simulink model "tqdtqr_rebuild_V3"  (R2021b)
settings: Solver=VariableStepAuto  StartTime=0.0  StopTime=10.0  RelTol=1e-3
undefined symbols (not defined in the file): ATQD_AfterTqMinGain_X_Deg, ATQD_APSCreepBaseTqD_X_kph, ATQD_APSCreepBaseTqD_Y_Deg, ATQD_APSCreepBaseTqR_X_kph, ATQD_APSCreepBaseTqR_Y_Deg, ATQD_APSCreepIterm_X_kph, ATQD_APSCreepIterm_Y_kph, ATQD_APSCreepPterm_X_kph, ATQD_APSCreepPterm_Y_kph, ATQD_APSDecReq_X_kph, ATQD_APSDecReq_Y_mps2, ATQD_APSDecReqCMD_X_kph, ATQD_APSDecReqTs_X_pct, ATQD_APSDecTimeGain_X_Deg, ATQD_APSDecTimeGain_Y_s, ATQD_APSReqLowSpd_X_Deg, ATQD_AutoHoldReleaseBPS_X_Deg, ATQD_AWDLoadTrqnsGain_X_kg, ATQD_AWDLoadTrqnsGain_Y_pct, ATQD_BOSEnBPSPosn_X_kph, ATQD_BOSMap_X_rpm, ATQD_BOSMap_Y_pct, ATQD_CreepBaseTqD_X_kph, ATQD_CreepBaseTqD_Y_Deg, ATQD_CreepBaseTqR_X_kph, ATQD_CreepBaseTqR_Y_Deg, ATQD_CreepBPSDisPosn_X_Deg, ATQD_CreepBPSDisPosnR_X_Deg, ATQD_CreepBPSEnPosn_X_Deg, ATQD_CreepBPSEnPosnR_X_Deg, ATQD_CreepDeltaTq_X_kph, ATQD_CreepIterm_X_kph, ATQD_CreepIterm_Y_kph, ATQD_CreepItermMaxLimit_X_pct, ATQD_CreepPreloadTime_X_kph, ATQD_CreepPreloadTq_X_kph, ATQD_CreepPreloadTq_Y_s, ATQD_CreepProtTq_X_Deg, ATQD_CreepPterm_X_kph, ATQD_CreepPterm_Y_kph, ATQD_CreepRrTqSpRat_X_rpm, ATQD_CreepRrTqSpRat_Y_Nm, ATQD_CreepTargetSpdD_X_pct, ATQD_CreepTargetSpdR_X_pct, ATQD_CreepUpLimitTq_X_rpm, ATQD_DecIneOPDHoldEnDelay_X_Deg, ATQD_DecIneOPDHoldEnDelay_Y_bar, ATQD_ECOTqMapD_X_rpm, ATQD_ECOTqMapD_Y_pct, ATQD_EMTqMapD_X_rpm, ATQD_EMTqMapD_Y_pct, ATQD_EOPDTqMapDCon_X_rpm, ATQD_EOPDTqMapDCon_Y_Deg, ATQD_EstInitVehWeight_X_c, ATQD_FAfterTqCMDGain_X_rpm, ATQD_FAfterTqCMDGain_Y_pct, ATQD_ForceLowSpd_X_Deg, ATQD_ForcePLimitSpd_X_Deg, ATQD_FrLossMAPLowV_X_rpm, ATQD_FrLossMAPLowV_Y_Nm ... (+949)
libraries: simulink x235, hcu_lib x208, tqr x63, tqd x6
(part 5 of 37)

== system tqdtqr_rebuild_V3/Main/Front//Rear first order input torque ==
  note: Front
  BInpConvert_outputs : Inport
  VTQD_AfterAvailableTqDemFr_Nm : Inport  Port=2
  VTQD_AfterAvailableTqDemRr_Nm : Inport  Port=3
  VTQR_FrFirstOrderOutTqDelay_Nm : Inport  Port=4
  VTQR_RrFirstOrderOutTqDelay_Nm : Inport  Port=5
  AND : Logic  AllPortsSameDT=off  OutDataTypeStr=boolean
  AND1 : Logic  AllPortsSameDT=off  OutDataTypeStr=boolean
  Bus Selector : BusSelector  OutputSignals=VTQR_RampTqCMDGain_c,VTQR_FrGearChange_flg,VTQR_FrTqZeroTrans_enum,VTQR_FrTqZeroTransLowBound_Nm,VTQR_FrTqZeroTransUpBound_Nm,VTQR_RrGearChange_flg,VTQR_RrTqZeroTrans_enum,VTQR_RrTqZeroTransLowBound_Nm,VTQR_RrTqZeroTransUpBound_Nm
  Constant{1,8,13..14} (4 alike) : Constant  Value=ZERO_FLOAT
  Constant10 : Constant  Value=ENUM_TQZEROTRANS_NOZEROTRANS
  Constant11 : Constant  Value=KTQR_NewRampArchSW_flg
  Constant12 : Constant  Value=ONE_FLOAT
  Constant2 : Constant  Value=KTQR_GearChangeTqSW_flg
  Constant3 : Constant  Value=ENUM_TQZEROTRANS_NOZEROTRANS
  Constant4 : Constant  Value=KTQR_NewRampArchSW_flg
  Constant5 : Constant  Value=ONE_FLOAT
  Constant6 : Constant  Value=ZERO_INT
  Constant7 : Constant  Value=ZERO_INT
  Constant9 : Constant  Value=KTQR_GearChangeTqSW_flg
  Product : Product
  Product1 : Product
  Relational Operator : RelationalOperator  Operator===  OutDataTypeStr=boolean  RndMeth=Simplest
  Relational Operator{1,3,6,8} (4 alike) : RelationalOperator  OutDataTypeStr=boolean  RndMeth=Simplest
  Relational Operator2 : RelationalOperator  Operator=<=  OutDataTypeStr=boolean  RndMeth=Simplest
  Relational Operator4 : RelationalOperator  Operator=<  OutDataTypeStr=boolean  RndMeth=Simplest
  Relational Operator5 : RelationalOperator  Operator===  OutDataTypeStr=boolean  RndMeth=Simplest
  Relational Operator7 : RelationalOperator  Operator=<=  OutDataTypeStr=boolean  RndMeth=Simplest
  Relational Operator9 : RelationalOperator  Operator=<  OutDataTypeStr=boolean  RndMeth=Simplest
  Switch{,1..2,7..9} (6 alike) : Switch  Criteria=u2 ~= 0
  Switch{3..6,10..13} (8 alike) : Switch  Criteria=u2 > Threshold
  VTQR_FrFirstOrderInpTq_Nm : Outport
  VTQR_RrFirstOrderInpTq_Nm : Outport  Port=2
  wires:
  Switch6/1 -> Switch1/1
  [VTQD_AfterAvailableTqDemFr_Nm] -> Relational Operator3/1
  [VTQR_FrTqZeroTransUpBound_Nm] -> Switch6/3
  [VTQD_AfterAvailableTqDemFr_Nm] -> Product/1
  Switch4/1 -> Product/2
  Constant7/1 -> Relational Operator4/2
  Relational Operator4/1 -> Switch6/2
  Constant5/1 -> Switch4/3
  Switch/1 -> Switch3/3
  [VTQD_AfterAvailableTqDemFr_Nm] -> Relational Operator4/1
  [VTQR_FrActRampTqDem_Nm] -> Switch2/3
  Constant6/1 -> Relational Operator3/2
  [VTQR_FrTqZeroTrans_enum] -> Relational Operator/1
  Relational Operator3/1 -> Switch5/2
  [VTQR_FrTqZeroTransLowBound_Nm] -> Switch5/3
  [VTQR_FrTqZeroTransUpBound_Nm] -> Switch5/1
  [VTQR_FrActRampTqDem_Nm] -> Switch/1
  Switch5/1 -> Switch2/1
  [VTQR_FrTqZeroTransLowBound_Nm] -> Switch6/1
  Constant2/1 -> AND/2
  [VTQR_FrTqZeroTransLowBound_Nm] -> Relational Operator2/2
  Relational Operator/1 -> Switch/2
  [VTQR_RampTqCMDGain_c] -> Switch4/1
  Switch1/1 -> Switch/3
  Constant4/1 -> Switch4/2
  [VTQR_FrGearChange_flg] -> AND/1
  AND/1 -> Switch3/2
  Product/1 -> [VTQR_FrActRampTqDem_Nm]  "VTQR_FrActRampTqDem_Nm"
  Constant1/1 -> Switch3/1
  [VTQR_FrFirstOrderOutTqDelay_Nm] -> Relational Operator2/1
  Relational Operator2/1 -> Switch2/2
  Switch2/1 -> Switch1/3
  [VTQR_FrTqZeroTransUpBound_Nm] -> Relational Operator1/2
  Switch3/1 -> [VTQR_FrFirstOrderInpTq_Nm]  "VTQR_FrFirstOrderInpTq_Nm"
  Constant3/1 -> Relational Operator/2
  Relational Operator1/1 -> Switch1/2
  [VTQR_FrFirstOrderOutTqDelay_Nm] -> Relational Operator1/1
  VTQD_AfterAvailableTqDemFr_Nm/1 -> [VTQD_AfterAvailableTqDemFr_Nm]
  VTQD_AfterAvailableTqDemRr_Nm/1 -> [VTQD_AfterAvailableTqDemRr_Nm]
  BInpConvert_outputs/1 -> Bus Selector/1
  Bus Selector/1 -> [VTQR_RampTqCMDGain_c]  "<VTQR_RampTqCMDGain_c>"
  Bus Selector/2 -> [VTQR_FrGearChange_flg]  "<VTQR_FrGearChange_flg>"
  Bus Selector/3 -> [VTQR_FrTqZeroTrans_enum]  "<VTQR_FrTqZeroTrans_enum>"
  Bus Selector/4 -> [VTQR_FrTqZeroTransLowBound_Nm]  "<VTQR_FrTqZeroTransLowBound_Nm>"
  Bus Selector/5 -> [VTQR_FrTqZeroTransUpBound_Nm]  "<VTQR_FrTqZeroTransUpBound_Nm>"
  [VTQR_RrGearChange_flg] -> AND1/1
  Relational Operator7/1 -> Switch9/2
  [VTQR_RrFirstOrderOutTqDelay_Nm] -> Relational Operator6/1
  [VTQR_RrTqZeroTrans_enum] -> Relational Operator5/1
  [VTQR_RrTqZeroTransUpBound_Nm] -> Relational Operator6/2
  Switch8/1 -> Switch7/3
  Constant10/1 -> Relational Operator5/2
  [VTQR_RrActRampTqDem_Nm] -> Switch9/3
  [VTQD_AfterAvailableTqDemRr_Nm] -> Relational Operator8/1
  Switch13/1 -> Switch8/1
  [VTQR_RrTqZeroTransUpBound_Nm] -> Switch13/3
  Relational Operator9/1 -> Switch13/2
  Constant12/1 -> Switch11/3
  Switch12/1 -> Switch9/1
  Constant14/1 -> Relational Operator9/2
  Constant13/1 -> Relational Operator8/2
  Relational Operator5/1 -> Switch7/2
  [VTQR_RrTqZeroTransLowBound_Nm] -> Switch13/1
  Constant9/1 -> AND1/2
  Constant8/1 -> Switch10/1
  [VTQR_RrTqZeroTransUpBound_Nm] -> Switch12/1
  Switch11/1 -> Product1/2
  [VTQR_RampTqCMDGain_c] -> Switch11/1
  [VTQD_AfterAvailableTqDemRr_Nm] -> Relational Operator9/1
  Relational Operator6/1 -> Switch8/2
  Relational Operator8/1 -> Switch12/2
  [VTQR_RrActRampTqDem_Nm] -> Switch7/1
  [VTQR_RrTqZeroTransLowBound_Nm] -> Switch12/3
  Constant11/1 -> Switch11/2
  [VTQD_AfterAvailableTqDemRr_Nm] -> Product1/1
  Switch10/1 -> [VTQR_RrFirstOrderInpTq_Nm]  "VTQR_RrFirstOrderInpTq_Nm"
  Switch7/1 -> Switch10/3
  Product1/1 -> [VTQR_RrActRampTqDem_Nm]  "VTQR_RrActRampTqDem_Nm"
  [VTQR_RrFirstOrderOutTqDelay_Nm] -> Relational Operator7/1
  AND1/1 -> Switch10/2
  [VTQR_RrTqZeroTransLowBound_Nm] -> Relational Operator7/2
  Switch9/1 -> Switch8/3
  Bus Selector/6 -> [VTQR_RrGearChange_flg]  "<VTQR_RrGearChange_flg>"
  Bus Selector/7 -> [VTQR_RrTqZeroTrans_enum]  "<VTQR_RrTqZeroTrans_enum>"
  Bus Selector/8 -> [VTQR_RrTqZeroTransLowBound_Nm]  "<VTQR_RrTqZeroTransLowBound_Nm>"
  Bus Selector/9 -> [VTQR_RrTqZeroTransUpBound_Nm]  "<VTQR_RrTqZeroTransUpBound_Nm>"
  [VTQR_FrFirstOrderInpTq_Nm] -> VTQR_FrFirstOrderInpTq_Nm/1
  [VTQR_RrFirstOrderInpTq_Nm] -> VTQR_RrFirstOrderInpTq_Nm/1
  VTQR_RrFirstOrderOutTqDelay_Nm/1 -> [VTQR_RrFirstOrderOutTqDelay_Nm]
  VTQR_FrFirstOrderOutTqDelay_Nm/1 -> [VTQR_FrFirstOrderOutTqDelay_Nm]

== system tqdtqr_rebuild_V3/Main/Front//Rear ramp enable judge ==
  note: Rear final torque
  note: Front final torque
  BSCPIn_outputs : Inport
  BInpConvert_outputs : Inport  Port=2
  VTQR_RampFEDUWhlTqReq_Nm : Inport  Port=3
  VTQD_AfterAvailableTqDemFr_Nm : Inport  Port=4
  VTQR_RampREDUWhlTqReq_Nm : Inport  Port=5
  VTQD_AfterAvailableTqDemRr_Nm : Inport  Port=6
  Add : Sum
  Add1 : Sum
  Bus Selector : BusSelector  OutputSignals=VVMC_ADASForceIdle_flg
  Bus Selector1 : BusSelector  OutputSignals=VTQD_LoSpdBrkCtrl_flg,VTQR_RampTqCMDGain_c,VTQR_ActFEDUTqUpLimit_Nm,VTQR_ActFEDUTqLowLimit_Nm,VTQD_FEDUWhlTqBRegen_Nm,VTQD_REDUWhlTqBRegen_Nm,VTQR_ActREDUTqUpLimit_Nm,VTQR_ActREDUTqLowLimit_Nm
  Constant : Constant  Value=TRUE
  Constant1 : Constant  Value=FALSE
  Constant10 : Constant  Value=ONE_INT
  Constant12 : Constant  Value=ONE_INT
  Constant13 : Constant  Value=KTQR_NewRampArchSW_flg
  Constant2 : Constant  Value=TRUE
  Constant3 : Constant  Value=FALSE
  Constant9 : Constant  Value=KTQR_NewRampArchSW_flg
  Logical Operator1 : Logic  Operator=OR  AllPortsSameDT=off  OutDataTypeStr=boolean
  Logical Operator2 : Logic  Operator=OR  AllPortsSameDT=off  OutDataTypeStr=boolean
  Product : Product
  Product1 : Product
  Saturation Dynamic : simulink/Discontinuities/Saturation Dynamic  OutMin=[]  OutMax=[]  OutDataTypeStr=Inherit: Same as second input  OutDataType=fixdt(1, 16)  OutScaling=2^-10  DoSatur=off
  Saturation Dynamic1 : simulink/Discontinuities/Saturation Dynamic  OutMin=[]  OutMax=[]  OutDataTypeStr=Inherit: Same as second input  OutDataType=fixdt(1, 16)  OutScaling=2^-10  DoSatur=off
  Switch{,1..3} (4 alike) : Switch  Criteria=u2 ~= 0
  Switch10 : Switch  Criteria=u2 > Threshold
  Switch11 : Switch  Criteria=u2 > Threshold
  VTQR_ActualFEDUWhlTqReq_Nm : Outport
  VTQR_NoABSFEDUWhlTqReq_Nm : Outport  Port=2
  VTQR_ActualREDUWhlTqReq_Nm : Outport  Port=3
  VTQR_NoABSREDUWhlTqReq_Nm : Outport  Port=4
  wires:
  Product/1 -> Switch/3
  Constant1/1 -> Switch2/1
  [VTQD_LoSpdBrkCtrl_flg] -> Logical Operator1/2
  Switch2/1 -> Switch/2  "VTQR_FrRampEnable_flg"
  [VINP_ADASForceIdle_flg] -> Logical Operator1/1
  Constant9/1 -> Switch10/2
  Switch10/1 -> Product/2
  [VTQR_ActFEDUTqLowLimit_Nm] -> Saturation Dynamic/3
  Switch/1 -> Saturation Dynamic/2
  Constant/1 -> Switch2/3
  [VTQR_ActFEDUTqUpLimit_Nm] -> Saturation Dynamic/1
  Add/1 -> VTQR_ActualFEDUWhlTqReq_Nm/1  "VTQR_ActualFEDUWhlTqReq_Nm"
  [VTQD_FEDUWhlTqBRegen_Nm] -> Add/1
  Logical Operator1/1 -> Switch2/2
  [VTQR_RampFEDUWhlTqReq_Nm] -> Switch/1
  [VTQR_RampTqCMDGain_c] -> Switch10/1
  Saturation Dynamic/1 -> Add/2, VTQR_NoABSFEDUWhlTqReq_Nm/1  "VTQR_NoABSFEDUWhlTqReq_Nm"
  [VTQD_AfterAvailableTqDemFr_Nm] -> Product/1
  BSCPIn_outputs/1 -> Bus Selector/1
  BInpConvert_outputs/1 -> Bus Selector1/1
  Bus Selector/1 -> [VINP_ADASForceIdle_flg]  "<VVMC_ADASForceIdle_flg>"
  Bus Selector1/1 -> [VTQD_LoSpdBrkCtrl_flg]  "<VTQD_LoSpdBrkCtrl_flg>"
  VTQR_RampFEDUWhlTqReq_Nm/1 -> [VTQR_RampFEDUWhlTqReq_Nm]
  VTQD_AfterAvailableTqDemFr_Nm/1 -> [VTQD_AfterAvailableTqDemFr_Nm]
  Bus Selector1/2 -> [VTQR_RampTqCMDGain_c]  "<VTQR_RampTqCMDGain_c>"
  Bus Selector1/3 -> [VTQR_ActFEDUTqUpLimit_Nm]  "<VTQR_ActFEDUTqUpLimit_Nm>"
  Bus Selector1/4 -> [VTQR_ActFEDUTqLowLimit_Nm]  "<VTQR_ActFEDUTqLowLimit_Nm>"
  Bus Selector1/5 -> [VTQD_FEDUWhlTqBRegen_Nm]  "<VTQD_FEDUWhlTqBRegen_Nm>"
  [VTQR_ActREDUTqLowLimit_Nm] -> Saturation Dynamic1/3
  [VINP_ADASForceIdle_flg] -> Logical Operator2/1
  [VTQD_AfterAvailableTqDemRr_Nm] -> Product1/1
  Switch1/1 -> Saturation Dynamic1/2
  Constant3/1 -> Switch3/1
  Product1/1 -> Switch1/3
  Constant2/1 -> Switch3/3
  [VTQR_RampREDUWhlTqReq_Nm] -> Switch1/1
  Saturation Dynamic1/1 -> VTQR_NoABSREDUWhlTqReq_Nm/1, Add1/2  "VTQR_NoABSREDUWhlTqReq_Nm"
  Switch11/1 -> Product1/2
  Constant13/1 -> Switch11/2
  [VTQR_RampTqCMDGain_c] -> Switch11/1
  [VTQR_ActREDUTqUpLimit_Nm] -> Saturation Dynamic1/1
  Logical Operator2/1 -> Switch3/2
  Switch3/1 -> Switch1/2  "VTQR_RrRampEnable_flg"
  Constant12/1 -> Switch11/3
  Add1/1 -> VTQR_ActualREDUWhlTqReq_Nm/1  "VTQR_ActualREDUWhlTqReq_Nm"
  [VTQD_LoSpdBrkCtrl_flg] -> Logical Operator2/2
  [VTQD_REDUWhlTqBRegen_Nm] -> Add1/1
  VTQR_RampREDUWhlTqReq_Nm/1 -> [VTQR_RampREDUWhlTqReq_Nm]
  VTQD_AfterAvailableTqDemRr_Nm/1 -> [VTQD_AfterAvailableTqDemRr_Nm]
  Bus Selector1/6 -> [VTQD_REDUWhlTqBRegen_Nm]  "<VTQD_REDUWhlTqBRegen_Nm>"
  Bus Selector1/7 -> [VTQR_ActREDUTqUpLimit_Nm]  "<VTQR_ActREDUTqUpLimit_Nm>"
  Bus Selector1/8 -> [VTQR_ActREDUTqLowLimit_Nm]  "<VTQR_ActREDUTqLowLimit_Nm>"
  Constant10/1 -> Switch10/3

== system tqdtqr_rebuild_V3/Main/Inverse and turn to motor torque ==
  note: Rear
  note: Front
  BSCPIn_outputs : Inport
  BInpConvert_outputs : Inport  Port=2
  VTQR_ActualFEDUWhlTqReq_Nm : Inport  Port=3
  VTQR_ActualREDUWhlTqReq_Nm : Inport  Port=4
  AND : Logic  AllPortsSameDT=off  OutDataTypeStr=boolean
  AND1 : Logic  AllPortsSameDT=off  OutDataTypeStr=boolean
  AND{2..5} (4 alike) : Logic  Inputs=3  AllPortsSameDT=off  OutDataTypeStr=boolean
  AND6 : Logic  Operator=OR  AllPortsSameDT=off  OutDataTypeStr=boolean
  AND7 : Logic  Operator=OR  AllPortsSameDT=off  OutDataTypeStr=boolean
  Bus Selector : BusSelector  OutputSignals=VVMC_ADASActive_flg
  Bus Selector1 : BusSelector  OutputSignals=VTQR_FrGearChange_flg,VTQD_PreLoadPreEn_flg,VTQD_PreLoadHold_flg,VTQD_GearActualPosn_enum,VTQR_RrGearChange_flg
  Constant : Constant  Value=KTQR_FrAbsoluteMTTqDir_flg
  Constant1 : Constant  Value=ENUM_GEARACTUALPOSN_R
  Constant{10..11,14,17} (4 alike) : Constant  Value=ONE_FLOAT
  Constant{8,12,15,18} (4 alike) : Constant  Value=ZERO_FLOAT
  Constant{9,13,16,19} (4 alike) : Constant  Value=MINUSONE_FLOAT
  Constant2 : Constant  Value=ENUM_GEARACTUALPOSN_R
  Constant21 : Constant  Value=KTQR_GearChangeTqSW_flg
  Constant23 : Constant  Value=KTQR_GearChangeTqDSW_flg
  Constant24 : Constant  Value=KTQR_GearChangeTqSW_flg
  Constant25 : Constant  Value=KTQR_GearChangeTqDSW_flg
  Constant26 : Constant  Value=KTQR_NewRampArchSW_flg
  Constant27 : Constant  Value=KTQR_NewRampArchSW_flg
  Constant3 : Constant  Value=KTQD_RrTMTotalGearRatio_gain
  Constant4 : Constant  Value=KTQR_RrAbsoluteMTTqDir_flg
  Constant5 : Constant  Value=KTQD_FrTMTotalGearRatio_gain
  Constant6 : Constant  Value=KTQR_FrTMGearEff_c
  Constant7 : Constant  Value=KTQR_RrTMGearEff_c
  Delay{,1..3} (4 alike) : Delay  DelayLength=1
  Divide : Product  Inputs=*//
  Divide1 : Product  Inputs=*//
  Equal : RelationalOperator  Operator===  OutDataTypeStr=boolean  RndMeth=Simplest
  Equal1 : RelationalOperator  Operator===  OutDataTypeStr=boolean  RndMeth=Simplest
  LiuZgSwitch1 : Switch  Criteria=u2 ~= 0  Threshold=0.5
      settings: AttributesFormatString=<%<Criteria>>
  LiuZgSwitch8 : Switch  Criteria=u2 ~= 0  Threshold=0.5
      settings: AttributesFormatString=<%<Criteria>>
  NOT{,1..3} (4 alike) : Logic  Operator=NOT  AllPortsSameDT=off  OutDataTypeStr=boolean
  Product{,1..3} (4 alike) : Product
  Relational Operator : RelationalOperator  Operator=>  OutDataTypeStr=boolean  RndMeth=Simplest
  Relational Operator1 : RelationalOperator  Operator=<  OutDataTypeStr=boolean  RndMeth=Simplest
  Relational Operator2 : RelationalOperator  Operator=<  OutDataTypeStr=boolean  RndMeth=Simplest
  Relational Operator3 : RelationalOperator  Operator=>  OutDataTypeStr=boolean  RndMeth=Simplest
  Switch{,1..3} (4 alike) : Switch  Criteria=u2 ~= 0
  Switch{4..9} (6 alike) : Switch  Criteria=u2 > Threshold
  VTQR_FrTMTqReq_Nm : Outport
  VTQR_RrTMTqReq_Nm : Outport  Port=2
  wires:
  AND7/1 -> Switch5/2
  [VTQR_FrGearChange_flg] -> Switch5/1
  [VTQR_ActualFEDUWhlTqReq_Nm] -> Product/2
  [VTQD_PreLoadPreEn_flg] -> AND3/2
  [VVMC_ADASActive_flg] -> AND7/2
  Switch8/1 -> Divide/1  "VTQR_InitFEDUWhlTqReq_Nm"
  [VTQD_PreLoadHold_flg] -> NOT1/1
  AND/1 -> LiuZgSwitch8/2
  Constant/1 -> AND/1
  NOT1/1 -> AND3/3
  Switch1/1 -> Product1/1
  Switch5/1 -> Switch1/2
  NOT/1 -> AND2/3
  LiuZgSwitch8/1 -> Switch8/3
  Product/1 -> LiuZgSwitch8/1
  AND3/1 -> Switch5/3
  Constant26/1 -> Switch8/2
  Product1/1 -> LiuZgSwitch8/3
  Constant21/1 -> Switch4/2
  [VTQR_ActualFEDUWhlTqReq_Nm] -> Switch8/1
  Equal/1 -> AND/2
  Switch4/1 -> Switch/2
  Switch/1 -> Product/1
  Constant11/1 -> Switch1/3
  [VTQD_GearActualPosn_enum] -> Equal/1
  Constant10/1 -> Switch/1
  Constant9/1 -> Switch/3
  Constant1/1 -> Equal/2
  Constant6/1 -> Divide/3
  Relational Operator1/1 -> AND3/1
  Relational Operator/1 -> AND2/1
  [VTQR_FrGearChange_flg] -> Switch4/1
  Delay1/1 -> Relational Operator1/1
  Divide/1 -> [VTQR_FrTMTqReq_Nm]  "VTQR_FrTMTqReq_Nm"
  AND2/1 -> Switch4/3
  [VTQR_ActualFEDUWhlTqReq_Nm] -> Product1/2
  Delay/1 -> Relational Operator/1
  [VTQR_FrTMTqReq_Nm] -> Delay/1
  Constant12/1 -> Relational Operator1/2
  Constant8/1 -> Relational Operator/2
  [VTQD_PreLoadHold_flg] -> NOT/1
  Constant23/1 -> AND7/1
  [VTQR_FrTMTqReq_Nm] -> Delay1/1
  Constant13/1 -> Switch1/1
  [VTQD_PreLoadPreEn_flg] -> AND2/2
  Constant5/1 -> Divide/2
  [VVMC_ADASActive_flg] -> AND6/2
  AND4/1 -> Switch7/3
  Switch6/1 -> Switch3/2
  [VTQR_ActualREDUWhlTqReq_Nm] -> Product3/2
  Delay2/1 -> Relational Operator2/1
  Constant24/1 -> Switch6/2
  Constant7/1 -> Divide1/3
  LiuZgSwitch1/1 -> Switch9/3
  [VTQR_RrTMTqReq_Nm] -> Delay2/1
  [VTQR_RrGearChange_flg] -> Switch7/1
  [VTQR_RrGearChange_flg] -> Switch6/1
  Constant27/1 -> Switch9/2
  [VTQD_GearActualPosn_enum] -> Equal1/1
  AND5/1 -> Switch6/3
  AND6/1 -> Switch7/2
  Switch7/1 -> Switch2/2
  [VTQD_PreLoadHold_flg] -> NOT3/1
  NOT3/1 -> AND5/3
  Constant15/1 -> Relational Operator2/2
  Constant19/1 -> Switch3/3
  Constant16/1 -> Switch2/1
  Product3/1 -> LiuZgSwitch1/1
  [VTQR_RrTMTqReq_Nm] -> Delay3/1
  Delay3/1 -> Relational Operator3/1
  Constant3/1 -> Divide1/2
  Constant2/1 -> Equal1/2
  AND1/1 -> LiuZgSwitch1/2
  [VTQD_PreLoadPreEn_flg] -> AND4/2
  NOT2/1 -> AND4/3
  Constant14/1 -> Switch2/3
  [VTQR_ActualREDUWhlTqReq_Nm] -> Switch9/1
  Equal1/1 -> AND1/2
  [VTQR_ActualREDUWhlTqReq_Nm] -> Product2/2
  Constant4/1 -> AND1/1
  [VTQD_PreLoadHold_flg] -> NOT2/1
  Product2/1 -> LiuZgSwitch1/3
  Constant25/1 -> AND6/1
  Constant18/1 -> Relational Operator3/2
  Switch2/1 -> Product2/1
  Divide1/1 -> [VTQR_RrTMTqReq_Nm]  "VTQR_RrTMTqReq_Nm"
  Constant17/1 -> Switch3/1
  Relational Operator3/1 -> AND5/1
  Switch3/1 -> Product3/1
  [VTQD_PreLoadPreEn_flg] -> AND5/2
  Relational Operator2/1 -> AND4/1
  Switch9/1 -> Divide1/1  "VTQR_InitREDUWhlTqReq_Nm"
  BSCPIn_outputs/1 -> Bus Selector/1
  BInpConvert_outputs/1 -> Bus Selector1/1
  Bus Selector1/1 -> [VTQR_FrGearChange_flg]  "<VTQR_FrGearChange_flg>"
  Bus Selector1/2 -> [VTQD_PreLoadPreEn_flg]  "<VTQD_PreLoadPreEn_flg>"
  Bus Selector1/3 -> [VTQD_PreLoadHold_flg]  "<VTQD_PreLoadHold_flg>"
  VTQR_ActualFEDUWhlTqReq_Nm/1 -> [VTQR_ActualFEDUWhlTqReq_Nm]
  VTQR_ActualREDUWhlTqReq_Nm/1 -> [VTQR_ActualREDUWhlTqReq_Nm]
  Bus Selector1/4 -> [VTQD_GearActualPosn_enum]  "<VTQD_GearActualPosn_enum>"
  Bus Selector/1 -> [VVMC_ADASActive_flg]  "<VVMC_ADASActive_flg>"
  Bus Selector1/5 -> [VTQR_RrGearChange_flg]  "<VTQR_RrGearChange_flg>"
  [VTQR_FrTMTqReq_Nm] -> VTQR_FrTMTqReq_Nm/1
  [VTQR_RrTMTqReq_Nm] -> VTQR_RrTMTqReq_Nm/1

== system tqdtqr_rebuild_V3/Main/Tq Coordination ==
  note: Determine coordination torque
  BSCPIn_outputs : Inport
  BInpConvert_outputs : Inport  Port=2
  VTQD_DriverWhlTqDem_Nm : Inport  Port=3
  Bus Selector : BusSelector  OutputSignals=VTQD_NoSuitbleGear_flg,VTQD_PreLoadHold_flg,VTQD_TotalWhlTqCapMot_Nm,VTQD_TotalWhlTqCapGen_Nm,VTQD_ForceIdleTqReq_Nm
  Bus Selector1 : BusSelector  OutputSignals=VVMC_ADASActive_flg,VVMC_ADASWhlTqReq_Nm,VVMC_CruzActive_flg,VVMC_CruzWhlTqReq_Nm,VVMC_MSAActive_flg,VVMC_MSAWhlTqReq_Nm,VVMC_APSActive_flg,VVMC_ADASForceIdle_flg
  Constant3 : Constant  Value=KTQD_NewTotalCapTqSW_flg
  Constant5 : Constant  Value=KTQD_DriverTqDemN_Nm
  Saturation Dynamic : simulink/Discontinuities/Saturation Dynamic  OutMin=[]  OutMax=[]  OutDataTypeStr=Inherit: Same as second input  OutDataType=fixdt(1, 16)  OutScaling=2^-10  DoSatur=off
  Switch{,1..6,8} (8 alike) : Switch  Criteria=u2 ~= 0
      settings: AttributesFormatString=%<Criteria>
  VTQD_CoordTqDem_Nm : Outport
  wires:
  [VTQD_TotalWhlTqCapMot_Nm] -> Saturation Dynamic/1
  [VTQD_TotalWhlTqCapGen_Nm] -> Saturation Dynamic/3
  Saturation Dynamic/1 -> Switch/1
  Constant3/1 -> Switch/2
  BInpConvert_outputs/1 -> Bus Selector/1
  BSCPIn_outputs/1 -> Bus Selector1/1
  Bus Selector1/1 -> [VVMC_ADASActive_flg]  "<VVMC_ADASActive_flg>"
  Bus Selector1/2 -> [VVMC_ADASWhlTqReq_Nm]  "<VVMC_ADASWhlTqReq_Nm>"
  Bus Selector1/3 -> [VVMC_CruzActive_flg]  "<VVMC_CruzActive_flg>"
  Bus Selector1/4 -> [VVMC_CruzWhlTqReq_Nm]  "<VVMC_CruzWhlTqReq_Nm>"
  Bus Selector1/5 -> [VVMC_MSAActive_flg]  "<VVMC_MSAActive_flg>"
  Bus Selector1/6 -> [VVMC_MSAWhlTqReq_Nm]  "<VVMC_MSAWhlTqReq_Nm>"
  Bus Selector1/7 -> [VVMC_APSActive_flg]  "<VVMC_APSActive_flg>"
  VTQD_DriverWhlTqDem_Nm/1 -> [VTQD_DriverWhlTqDem_Nm]
  Bus Selector1/8 -> [VINP_ADASForceIdle_flg]  "<VVMC_ADASForceIdle_flg>"
  Bus Selector/2 -> [VTQD_PreLoadHold_flg]  "<VTQD_PreLoadHold_flg>"
  Bus Selector/3 -> [VTQD_TotalWhlTqCapMot_Nm]  "<VTQD_TotalWhlTqCapMot_Nm>"
  Bus Selector/4 -> [VTQD_TotalWhlTqCapGen_Nm]  "<VTQD_TotalWhlTqCapGen_Nm>"
  Switch/1 -> [VTQD_CoordTqDem_Nm]  "VTQD_CoordTqDem_Nm"
  Bus Selector/1 -> [VTQD_NoSuitbleGear_flg]  "<VTQD_NoSuitbleGear_flg>"
  [VTQD_NoSuitbleGear_flg] -> Switch1/2
  Switch1/1 -> [VTQD_WhlTqReqMerge_Nm]
  Constant5/1 -> Switch1/1
  Switch8/1 -> Switch1/3
  [VINP_ADASForceIdle_flg] -> Switch8/2
  Switch2/1 -> Switch8/3
  [VVMC_ADASActive_flg] -> Switch2/2
  [VTQD_PreLoadHold_flg] -> Switch3/2
  Switch3/1 -> Switch2/1
  [VVMC_ADASWhlTqReq_Nm] -> Switch3/3
  [VTQD_DriverWhlTqDem_Nm] -> Switch3/1
  Switch4/1 -> Switch2/3
  [VVMC_MSAActive_flg] -> Switch5/2
  [VVMC_MSAWhlTqReq_Nm] -> Switch5/1
  [VVMC_CruzWhlTqReq_Nm] -> Switch4/1
  [VVMC_CruzActive_flg] -> Switch4/2
  Switch5/1 -> Switch4/3
  Switch6/1 -> Switch5/3
  [VVMC_APSActive_flg] -> Switch6/2
  [VTQD_DriverWhlTqDem_Nm] -> Switch6/1
  [VTQD_DriverWhlTqDem_Nm] -> Switch6/3
  [VTQD_WhlTqReqMerge_Nm] -> Saturation Dynamic/2
  [VTQD_WhlTqReqMerge_Nm] -> Switch/3
  [VTQD_CoordTqDem_Nm] -> VTQD_CoordTqDem_Nm/1
  Bus Selector/5 -> [VTQD_ForceIdleTqReq_Nm]  "<VTQD_ForceIdleTqReq_Nm>"
  [VTQD_ForceIdleTqReq_Nm] -> Switch8/1

== system tqdtqr_rebuild_V3/Main/Tq Distribution ==
  note: Calculate Fr/Rr demand torque
  BSCPIn_outputs : Inport
  BInpConvert_outputs : Inport  Port=2
  TqCoordination_outputs : Inport  Port=3
  AND : Logic  Inputs=4  AllPortsSameDT=off  OutDataTypeStr=boolean
  AND1 : Logic  Inputs=4  AllPortsSameDT=off  OutDataTypeStr=boolean
  AND11 : Logic  Inputs=3  AllPortsSameDT=off  OutDataTypeStr=boolean
  AND{8..9,12,14} (4 alike) : Logic  AllPortsSameDT=off  OutDataTypeStr=boolean
  AND13 : Logic  Inputs=3  AllPortsSameDT=off  OutDataTypeStr=boolean
  Add : Sum
  Add1 : Sum  Inputs=+-
  Add2 : Sum
  Add3 : Sum  Inputs=+-
  Bus Selector : BusSelector  OutputSignals=VINP_RearAxlTrqReqDrv_Nm,VPMM_DrivetrainSelect_enum,VINP_RrPTCSActive_flg,VINP_FrPTCSActive_flg,VINP_FrntAxlTrqReqDrv_Nm
  Bus Selector1 : BusSelector  OutputSignals=VTQD_RockModePedTqFr_Nm,VTQD_RockModeTqLim_flg,VTQD_FrPreloadTq_Nm,VTQD_PreLoadHold_flg,VTQD_RockModePedTqRr_Nm,VTQD_RrPreloadTq_Nm,VTQD_NewDistFrWhlTq_Nm,VTQD_NewDistRrWhlTq_Nm,VTQD_FrEDUSpRat_rat,VTQD_RrEDUSpRat_rat
  Constant27 : Constant  Value=KTQD_RocModeTqCtrlSW_flg  VectorParams1D=off  SampleTime=-1
  Constant28 : Constant  Value=KTQD_RocModeTqCtrlSW_flg  VectorParams1D=off  SampleTime=-1
  Constant3 : Constant  Value=ENUM_DRIVETRAIN_AWD  VectorParams1D=off  SampleTime=-1
  Constant{34,37..38,41} (4 alike) : Constant  Value=KTQD_NewPrelaodSW_flg  VectorParams1D=off  SampleTime=-1
  Constant35 : Constant  Value=KTQD_NewWhlTqDistSW_flg  VectorParams1D=off  SampleTime=-1
  Constant36 : Constant  Value=KTQD_NewTotalCapTqSW_flg  VectorParams1D=off  SampleTime=-1
  Constant39 : Constant  Value=KTQD_NewWhlTqDistSW_flg  VectorParams1D=off  SampleTime=-1
  Constant4 : Constant  Value=ZERO_FLOAT  VectorParams1D=off  SampleTime=-1
  Constant40 : Constant  Value=KTQD_NewTotalCapTqSW_flg  VectorParams1D=off  SampleTime=-1
  Constant5 : Constant  Value=KTQD_RrTCSCompensateSW_flg  VectorParams1D=off  SampleTime=-1
  Constant6 : Constant  Value=ENUM_DRIVETRAIN_AWD  VectorParams1D=off  SampleTime=-1
  Constant7 : Constant  Value=ZERO_FLOAT  VectorParams1D=off  SampleTime=-1
  Constant8 : Constant  Value=KTQD_FrTCSCompensateSW_flg  VectorParams1D=off  SampleTime=-1
  Equal3 : RelationalOperator  Operator===  OutDataTypeStr=boolean  RndMeth=Simplest
  Equal4 : RelationalOperator  Operator===  OutDataTypeStr=boolean  RndMeth=Simplest
  NOT : Logic  Operator=NOT  AllPortsSameDT=off  OutDataTypeStr=boolean
  NOT2 : Logic  Operator=NOT  AllPortsSameDT=off  OutDataTypeStr=boolean
  Product1 : Product
  Product4 : Product
  Saturation : Saturate  UpperLimit=KTQD_TCSCompUpLimit_Nm  LowerLimit=ZERO_FLOAT
      settings: AttributesFormatString=%<UpperLimit>
  Saturation1 : Saturate  UpperLimit=KTQD_TCSCompUpLimit_Nm  LowerLimit=ZERO_FLOAT
      settings: AttributesFormatString=%<UpperLimit>
  Switch{,1,8..9,11..14} (8 alike) : Switch  Criteria=u2 ~= 0
      settings: AttributesFormatString=%<Criteria>
  VTQD_CoordWhlTqDemFr_Nm : Outport
  VTQD_CoordWhlTqDemRr_Nm : Outport  Port=2
  VTQD_CoordTqDemFr_Nm : Outport  Port=3
  VTQD_CoordTqDemRr_Nm : Outport  Port=4
  wires:
  BSCPIn_outputs/1 -> Bus Selector/1
  BInpConvert_outputs/1 -> Bus Selector1/1
  [VTQD_FrEDUSpRat_rat] -> Product4/1
  Constant36/1 -> AND11/2
  Constant34/1 -> AND12/2
  Constant35/1 -> AND11/3
  Switch1/1 -> Saturation1/1
  [VTQD_RockModeTqLim_flg] -> AND8/1
  Switch8/1 -> Add2/2, [VTQD_CoordTqDemFr_Nm]  "VTQD_CoordTqDemFr_Nm"
  [VTQD_CoordTqDem_Nm] -> Product4/2
  [VTQD_RockModePedTqFr_Nm] -> Switch8/1
  AND8/1 -> Switch8/2
  [VINP_RrPTCSActive_flg] -> AND1/2
  Constant8/1 -> AND1/4
  Constant7/1 -> Switch1/3
  Equal4/1 -> AND1/1
  [VTQD_CoordTqDemRr_Nm] -> Add3/1
  [VINP_FrPTCSActive_flg] -> NOT/1
  [VTQD_PreLoadHold_flg] -> AND12/1
  AND1/1 -> Switch1/2
  [VPMM_DrivetrainSelect_enum] -> Equal4/1
  Saturation1/1 -> Add2/1  "VTQD_FrTCSCompensateTq_Nm"
  AND12/1 -> Switch11/2
  Constant6/1 -> Equal4/2
  [VTQD_NewDistFrWhlTq_Nm] -> Switch12/1
  Switch11/1 -> Switch12/3
  NOT/1 -> AND1/3
  AND11/1 -> Switch12/2
  Add3/1 -> Switch1/1
  Constant27/1 -> AND8/2
  [VTQD_FrPreloadTq_Nm] -> Switch11/1
  [VINP_RearAxlTrqReqDrv_Nm] -> Add3/2
  Switch12/1 -> Switch8/3
  Product4/1 -> Switch11/3
  Constant37/1 -> AND11/1
  Constant39/1 -> AND13/3
  Constant40/1 -> AND13/2
  AND13/1 -> Switch14/2
  Product1/1 -> Switch13/3
  AND14/1 -> Switch13/2
  [VTQD_RrPreloadTq_Nm] -> Switch13/1
  Switch13/1 -> Switch14/3
  Switch9/1 -> Add/2, [VTQD_CoordTqDemRr_Nm]  "VTQD_CoordTqDemRr_Nm"
  Constant38/1 -> AND14/2
  Constant41/1 -> AND13/1
  [VTQD_NewDistRrWhlTq_Nm] -> Switch14/1
  Switch/1 -> Saturation/1
  Constant3/1 -> Equal3/2
  AND9/1 -> Switch9/2
  AND/1 -> Switch/2
  Constant28/1 -> AND9/2
  [VTQD_RockModeTqLim_flg] -> AND9/1
  NOT2/1 -> AND/3
  [VTQD_CoordTqDemFr_Nm] -> Add1/1
  Saturation/1 -> Add/1  "VTQD_RrTCSCompensateTq_Nm"
  [VPMM_DrivetrainSelect_enum] -> Equal3/1
  Add/1 -> [VTQD_CoordWhlTqDemRr_Nm]  "VTQD_CoordWhlTqDemRr_Nm"
  Constant5/1 -> AND/4
  Constant4/1 -> Switch/3
  Add1/1 -> Switch/1
  [VTQD_PreLoadHold_flg] -> AND14/1
  [VINP_RrPTCSActive_flg] -> NOT2/1
  Switch14/1 -> Switch9/3
  [VTQD_RrEDUSpRat_rat] -> Product1/1
  [VTQD_CoordTqDem_Nm] -> Product1/2
  [VINP_FrntAxlTrqReqDrv_Nm] -> Add1/2
  [VTQD_RockModePedTqRr_Nm] -> Switch9/1
  [VINP_FrPTCSActive_flg] -> AND/2
  Equal3/1 -> AND/1
  Bus Selector/1 -> [VINP_RearAxlTrqReqDrv_Nm]  "<VINP_RearAxlTrqReqDrv_Nm>"
  Bus Selector/2 -> [VPMM_DrivetrainSelect_enum]  "<VPMM_DrivetrainSelect_enum>"
  Bus Selector/3 -> [VINP_RrPTCSActive_flg]  "<VINP_RrPTCSActive_flg>"
  Bus Selector/4 -> [VINP_FrPTCSActive_flg]  "<VINP_FrPTCSActive_flg>"
  Bus Selector1/1 -> [VTQD_RockModePedTqFr_Nm]  "<VTQD_RockModePedTqFr_Nm>"
  Bus Selector1/2 -> [VTQD_RockModeTqLim_flg]  "<VTQD_RockModeTqLim_flg>"
  Bus Selector1/3 -> [VTQD_FrPreloadTq_Nm]  "<VTQD_FrPreloadTq_Nm>"
  Bus Selector1/4 -> [VTQD_PreLoadHold_flg]  "<VTQD_PreLoadHold_flg>"
  Bus Selector/5 -> [VINP_FrntAxlTrqReqDrv_Nm]  "<VINP_FrntAxlTrqReqDrv_Nm>"
  Bus Selector1/5 -> [VTQD_RockModePedTqRr_Nm]  "<VTQD_RockModePedTqRr_Nm>"
  Bus Selector1/6 -> [VTQD_RrPreloadTq_Nm]  "<VTQD_RrPreloadTq_Nm>"
  Add2/1 -> [VTQD_CoordWhlTqDemFr_Nm]  "VTQD_CoordWhlTqDemFr_Nm"
  Bus Selector1/7 -> [VTQD_NewDistFrWhlTq_Nm]  "<VTQD_NewDistFrWhlTq_Nm>"
  Bus Selector1/8 -> [VTQD_NewDistRrWhlTq_Nm]  "<VTQD_NewDistRrWhlTq_Nm>"
  TqCoordination_outputs/1 -> [VTQD_CoordTqDem_Nm]
  Bus Selector1/9 -> [VTQD_FrEDUSpRat_rat]  "<VTQD_FrEDUSpRat_rat>"
  Bus Selector1/10 -> [VTQD_RrEDUSpRat_rat]  "<VTQD_RrEDUSpRat_rat>"
  [VTQD_CoordWhlTqDemFr_Nm] -> VTQD_CoordWhlTqDemFr_Nm/1
  [VTQD_CoordWhlTqDemRr_Nm] -> VTQD_CoordWhlTqDemRr_Nm/1
  [VTQD_CoordTqDemFr_Nm] -> VTQD_CoordTqDemFr_Nm/1
  [VTQD_CoordTqDemRr_Nm] -> VTQD_CoordTqDemRr_Nm/1

== system tqdtqr_rebuild_V3/Output_Convert/Avaliable Torque ==
  note: Avaiable Torque for B-type Regen
  note: A-regen activation judgment
  BSCPIn_outputs : Inport
  BInpConvert_outputs : Inport  Port=2
  BMain_outputs : Inport  Port=3
  VTQD_DriverWhlTqDemFr_Nm : Inport  Port=4
  VTQD_DriverWhlTqDemRr_Nm : Inport  Port=5
  Bus Selector : BusSelector  OutputSignals=task_time_s,VVMC_ADASActive_flg,VINP_FrRegenAvailTq_Nm,VINP_RrRegenAvailTq_Nm,VINP_HVBattSOC_pct,VPMM_DrivetrainSelect_enum
  Bus Selector1 : BusSelector  OutputSignals=VTQD_TqSourceFr_enum,VTQD_TqSourceRr_enum,VTQD_CreepEnable_flg,VTQD_WhlTqCapGenFr_Nm,VTQD_WhlTqCapGenRr_Nm,VTQD_VehActSpd_kph,VTQD_GearActualPosn_enum
  Bus Selector2 : BusSelector  OutputSignals=VTQD_DriverWhlTqDem_Nm
  Constant{,4,7,37,44} (5 alike) : Constant  Value=FALSE
  Constant1 : Constant  Value=ENUM_TQSOURCE_CC
  Constant10 : Constant  Value=ENUM_TQSOURCE_APS
  Constant11 : Constant  Value=ENUM_TQSOURCE_CC
  Constant12 : Constant  Value=ENUM_TQSOURCE_APS
  Constant13 : Constant  Value=ENUM_TQSOURCE_ADAS
  Constant{14,17,20,33,48} (5 alike) : Constant  Value=ZERO_FLOAT
  Constant15 : Constant  Value=KTQD_AvailBrkRgnTqSpd_kph
  Constant18 : Constant  Value=KTQD_AvailBrkRgnTqSpd_kph
  Constant{3,6,8,38,45} (5 alike) : Constant  Value=TRUE
  Constant34 : Constant  Value=KTQD_AvailBRgnTqVSOC_pct
  Constant35 : Constant  Value=ENUM_GEARACTUALPOSN_N
  Constant36 : Constant  Value=ENUM_GEARACTUALPOSN_P
  Constant39 : Constant  Value=ENUM_DRIVETRAIN_RWD
  Constant40 : Constant  Value=ENUM_DRIVETRAIN_RWD
  Constant41 : Constant  Value=KTQD_BRgnPermDisDelay_s
  Constant42 : Constant  Value=ENUM_GEARACTUALPOSN_N
  Constant43 : Constant  Value=ENUM_GEARACTUALPOSN_P
  Constant46 : Constant  Value=ENUM_DRIVETRAIN_FWD
  Constant47 : Constant  Value=KTQD_BRgnPermDisDelay_s
  Constant49 : Constant  Value=KTQD_AvailBRgnTqVSOC_pct
  Constant50 : Constant  Value=ENUM_DRIVETRAIN_FWD
  Constant9 : Constant  Value=ENUM_TQSOURCE_ADAS
  Data Type Conversion : DataTypeConversion  OutDataTypeStr=single
  Data Type Conversion1 : DataTypeConversion  OutDataTypeStr=single
  DelayEnable : hcu_lib/Basic_Blocks/DelayEnable
  DelayEnable1 : hcu_lib/Basic_Blocks/DelayEnable
  Equal{,1..5,10..17} (14 alike) : RelationalOperator  Operator===  OutDataTypeStr=boolean  RndMeth=Simplest
  Gain : Gain  Gain=KTQD_FrTMTotalGearRatio_gain
  Gain1 : Gain  Gain=KTQD_RrTMTotalGearRatio_gain
  If : If  IfExpression=u1 ~= 0
  If Action Subsystem1 : tqd/TQD/TorqueDemand/TorqueModule/AvaliableTqLimit/If Action Subsystem1  SystemSampleTime=-1  VariantActivationTime=update diagram  Latency=0  AutoFrameSizeCalculation=off
  If Action Subsystem2 : tqd/TQD/TorqueDemand/TorqueModule/AvaliableTqLimit/If Action Subsystem2  SystemSampleTime=-1  VariantActivationTime=update diagram  Latency=0  AutoFrameSizeCalculation=off
  Logical Operator : Logic  Operator=OR  Inputs=7  AllPortsSameDT=off  OutDataTypeStr=boolean
  Logical Operator1 : Logic  AllPortsSameDT=off  OutDataTypeStr=boolean
  Logical Operator2 : Logic  Operator=NOT  AllPortsSameDT=off  OutDataTypeStr=boolean
  Max : MinMax  Function=max  Inputs=2
  Max1 : MinMax  Function=max  Inputs=2
  Merge : Merge
  Merge1 : Merge
  OR2 : Logic  Operator=OR  Inputs=3  AllPortsSameDT=off  OutDataTypeStr=boolean
  OR{3..6} (4 alike) : Logic  Operator=OR  AllPortsSameDT=off  OutDataTypeStr=boolean
  OR7 : Logic  Operator=OR  Inputs=3  AllPortsSameDT=off  OutDataTypeStr=boolean
  Relational Operator : RelationalOperator  Operator=<  OutDataTypeStr=boolean  RndMeth=Simplest
  Relational Operator1 : RelationalOperator  Operator=<=  OutDataTypeStr=boolean  RndMeth=Simplest
  Relational Operator2 : RelationalOperator  Operator=<=  OutDataTypeStr=boolean  RndMeth=Simplest
  Relational Operator{3..6} (4 alike) : RelationalOperator  OutDataTypeStr=boolean  RndMeth=Simplest
  Switch{,1,11..12} (4 alike) : Switch  Criteria=u2 > Threshold
  Switch2 : Switch  Criteria=u2 ~= 0
  Switch3 : Switch  Criteria=u2 ~= 0
  Switch4 : Switch  Criteria=u2 ~= 0
  VTQD_ARegenActive_flg : Outport
  VTQD_FrEDUAvailBrkRgnTq_Nm : Outport  Port=2
  VTQD_RrEDUAvailBrkRgnTq_Nm : Outport  Port=3
  VTQD_FrRgnDecrSta_flg : Outport  Port=4
  VTQD_RrRgnDecrSta_flg : Outport  Port=5
  VTQD_FrRgnPermSta_flg : Outport  Port=6
  VTQD_RrRgnPermSta_flg : Outport  Port=7
  wires:
  Logical Operator/1 -> Logical Operator2/1
  [VTQD_FrEDUAvailBrkRgnTq_Nm] -> Relational Operator3/1
  OR4/1 -> Switch11/2
  [VPMM_DrivetrainSelect_enum] -> Equal13/1
  [task_time_s] -> DelayEnable/3
  Constant20/1 -> Switch4/1
  Constant47/1 -> DelayEnable1/2
  Constant13/1 -> Equal4/2
  Constant45/1 -> Switch12/3
  Max1/1 -> Switch4/3
  Constant10/1 -> Equal2/2
  [VTQD_GearActualPosn_enum] -> Equal15/1
  [VTQD_DriverWhlTqDemRr_Nm] -> If Action Subsystem1/4
  [VPMM_DrivetrainSelect_enum] -> Equal12/1
  Constant9/1 -> Equal1/2
  Constant6/1 -> Switch1/3
  Constant18/1 -> Relational Operator2/2
  OR6/1 -> Switch12/2
  Constant44/1 -> Switch12/1
  Constant46/1 -> Equal16/2
  OR5/1 -> DelayEnable1/1
  Switch2/1 -> [VTQD_ARegenActive_flg]  "VTQD_ARegenActive_flg"
  [VVMC_ADASActive_flg] -> If Action Subsystem1/5
  [task_time_s] -> DelayEnable1/3
  Equal13/1 -> OR4/2
  Equal14/1 -> OR5/1
  Equal11/1 -> OR3/2
  [VTQD_AvailTqNoARgnFr_Nm] -> Merge/2
  Constant1/1 -> Equal/2
  DelayEnable/1 -> OR4/1
  Switch4/1 -> Data Type Conversion1/1
  OR3/1 -> DelayEnable/1
  Constant34/1 -> Relational Operator4/2
  [VTQD_GearActualPosn_enum] -> Equal11/1
  Constant41/1 -> DelayEnable/2
  [VTQD_RrEDUAvailBrkRgnTq_Nm] -> Relational Operator5/1
  Relational Operator6/1 -> OR7/2
  DelayEnable1/1 -> OR6/1
  [VPMM_DrivetrainSelect_enum] -> Equal17/1
  Constant40/1 -> Equal13/2
  Constant38/1 -> Switch11/3
  Relational Operator3/1 -> OR2/1
  [VTQD_TqSourceFr_enum] -> Equal/1
  [VTQD_GearActualPosn_enum] -> Equal10/1
  Constant37/1 -> Switch11/1
  Max/1 -> Switch3/3
  [VTQD_CreepEnable_flg] -> Logical Operator/7
  Equal10/1 -> OR3/1
  Constant35/1 -> Equal10/2
  [VTQD_AvailTqWithARgnFr_Nm] -> Merge/1
  Relational Operator4/1 -> OR2/2
  Constant33/1 -> Relational Operator3/2
  If/2 -> If Action Subsystem2/Action
  Constant/1 -> Switch/1
  Constant3/1 -> Switch/3
  [VINP_RrRegenAvailTq_Nm] -> Gain1/1
  Switch3/1 -> Data Type Conversion/1
  [VTQD_WhlTqCapGenFr_Nm] -> If Action Subsystem1/1
  [VTQD_DriverWhlTqDemFr_Nm] -> If Action Subsystem1/3
  If/1 -> If Action Subsystem1/Action
  Constant50/1 -> Equal17/2
  Logical Operator1/1 -> Switch2/2
  Relational Operator5/1 -> OR7/1
  Relational Operator1/1 -> Switch3/2
  Constant17/1 -> Switch3/1
  Equal15/1 -> OR5/2
  Equal1/1 -> Logical Operator/2
  Relational Operator/1 -> Logical Operator1/2
  [VTQD_TqSourceFr_enum] -> Equal2/1
  [VTQD_AvailTqWithARgnRr_Nm] -> Merge1/1
  [VTQD_TqSourceRr_enum] -> Equal3/1
  [VTQD_TqSourceRr_enum] -> Equal4/1
  [VTQD_TqSourceRr_enum] -> Equal5/1
  Equal4/1 -> Logical Operator/5
  Equal5/1 -> Logical Operator/6
  If Action Subsystem1/2 -> [VTQD_AvailTqWithARgnRr_Nm]
  Data Type Conversion/1 -> [VTQD_FrEDUAvailBrkRgnTq_Nm]  "VTQD_FrEDUAvailBrkRgnTq_Nm"
  [VTQD_DriverWhlTqDem_Nm] -> Relational Operator/1
  Constant15/1 -> Relational Operator1/2
  [VINP_HVBattSOC_pct] -> Relational Operator4/1
  Constant12/1 -> Equal5/2
  Gain/1 -> Max/1
  [VTQD_VehActSpd_kph] -> Relational Operator1/1
  If Action Subsystem2/1 -> [VTQD_AvailTqNoARgnFr_Nm]
  Data Type Conversion1/1 -> [VTQD_RrEDUAvailBrkRgnTq_Nm]  "VTQD_RrEDUAvailBrkRgnTq_Nm"
  Equal16/1 -> OR6/2
  Logical Operator2/1 -> Logical Operator1/1
  Equal3/1 -> Logical Operator/4
  Merge/1 -> Max/2
  OR7/1 -> Switch1/2
  If Action Subsystem1/1 -> [VTQD_AvailTqWithARgnFr_Nm]
  Gain1/1 -> Max1/1
  Equal2/1 -> Logical Operator/3
  [VTQD_TqSourceFr_enum] -> Equal1/1
  OR2/1 -> Switch/2
  [VTQD_AvailTqNoARgnRr_Nm] -> Merge1/2
  Relational Operator2/1 -> Switch4/2
  Constant42/1 -> Equal14/2
  [VINP_HVBattSOC_pct] -> Relational Operator6/1
  [VTQD_WhlTqCapGenRr_Nm] -> If Action Subsystem1/2
  Constant48/1 -> Relational Operator5/2
  Equal12/1 -> OR2/3
  Constant8/1 -> Switch2/1
  [VTQD_GearActualPosn_enum] -> Equal14/1
  [VTQD_WhlTqCapGenRr_Nm] -> If Action Subsystem2/2
  Merge1/1 -> Max1/2
  Constant4/1 -> Switch1/1
  If Action Subsystem2/2 -> [VTQD_AvailTqNoARgnRr_Nm]
  Constant36/1 -> Equal11/2
  [VPMM_DrivetrainSelect_enum] -> Equal16/1
  Constant49/1 -> Relational Operator6/2
  Constant14/1 -> Relational Operator/2
  [VTQD_ARegenActive_flg] -> If/1
  [VTQD_WhlTqCapGenFr_Nm] -> If Action Subsystem2/1
  Equal17/1 -> OR7/3
  Equal/1 -> Logical Operator/1
  Constant11/1 -> Equal3/2
  Constant43/1 -> Equal15/2
  Constant7/1 -> Switch2/3
  [VTQD_VehActSpd_kph] -> Relational Operator2/1
  [VINP_FrRegenAvailTq_Nm] -> Gain/1
  Constant39/1 -> Equal12/2
  BSCPIn_outputs/1 -> Bus Selector/1
  BInpConvert_outputs/1 -> Bus Selector1/1
  BMain_outputs/1 -> Bus Selector2/1
  Bus Selector1/1 -> [VTQD_TqSourceFr_enum]  "<VTQD_TqSourceFr_enum>"
  Bus Selector1/2 -> [VTQD_TqSourceRr_enum]  "<VTQD_TqSourceRr_enum>"
  Bus Selector1/3 -> [VTQD_CreepEnable_flg]  "<VTQD_CreepEnable_flg>"
  Bus Selector2/1 -> [VTQD_DriverWhlTqDem_Nm]  "<VTQD_DriverWhlTqDem_Nm>"
  Bus Selector1/4 -> [VTQD_WhlTqCapGenFr_Nm]  "<VTQD_WhlTqCapGenFr_Nm>"
  Bus Selector1/5 -> [VTQD_WhlTqCapGenRr_Nm]  "<VTQD_WhlTqCapGenRr_Nm>"
  VTQD_DriverWhlTqDemFr_Nm/1 -> [VTQD_DriverWhlTqDemFr_Nm]
  VTQD_DriverWhlTqDemRr_Nm/1 -> [VTQD_DriverWhlTqDemRr_Nm]
  Bus Selector/2 -> [VVMC_ADASActive_flg]  "<VVMC_ADASActive_flg>"
  Bus Selector/3 -> [VINP_FrRegenAvailTq_Nm]  "<VINP_FrRegenAvailTq_Nm>"
  Bus Selector1/6 -> [VTQD_VehActSpd_kph]  "<VTQD_VehActSpd_kph>"
  Bus Selector/4 -> [VINP_RrRegenAvailTq_Nm]  "<VINP_RrRegenAvailTq_Nm>"
  Bus Selector/5 -> [VINP_HVBattSOC_pct]  "<VINP_HVBattSOC_pct>"
  Bus Selector/6 -> [VPMM_DrivetrainSelect_enum]  "<VPMM_DrivetrainSelect_enum>"
  Bus Selector/1 -> [task_time_s]  "<task_time_s>"
  Bus Selector1/7 -> [VTQD_GearActualPosn_enum]  "<VTQD_GearActualPosn_enum>"
  Switch/1 -> [VTQD_FrRgnDecrSta_flg]  "VTQD_FrRgnDecrSta_flg"
  Switch1/1 -> [VTQD_RrRgnDecrSta_flg]  "VTQD_RrRgnDecrSta_flg"
  Switch11/1 -> [VTQD_FrRgnPermSta_flg]  "VTQD_FrRgnPermSta_flg"
  Switch12/1 -> [VTQD_RrRgnPermSta_flg]  "VTQD_RrRgnPermSta_flg"
  [VTQD_ARegenActive_flg] -> VTQD_ARegenActive_flg/1
  [VTQD_FrEDUAvailBrkRgnTq_Nm] -> VTQD_FrEDUAvailBrkRgnTq_Nm/1
  [VTQD_RrEDUAvailBrkRgnTq_Nm] -> VTQD_RrEDUAvailBrkRgnTq_Nm/1
  [VTQD_FrRgnDecrSta_flg] -> VTQD_FrRgnDecrSta_flg/1
  [VTQD_RrRgnDecrSta_flg] -> VTQD_RrRgnDecrSta_flg/1
  [VTQD_FrRgnPermSta_flg] -> VTQD_FrRgnPermSta_flg/1
  [VTQD_RrRgnPermSta_flg] -> VTQD_RrRgnPermSta_flg/1
